simulink subsystem "DCDC_Generator"  (R2024a)
settings: Solver=VariableStepAuto  StartTime=0.0  StopTime=10.0  RelTol=1e-3
undefined symbols (not defined in the file): eta_conv, eta_rect, R_rect, V_drop
settings Model: Creator=User  LastModifiedBy=User

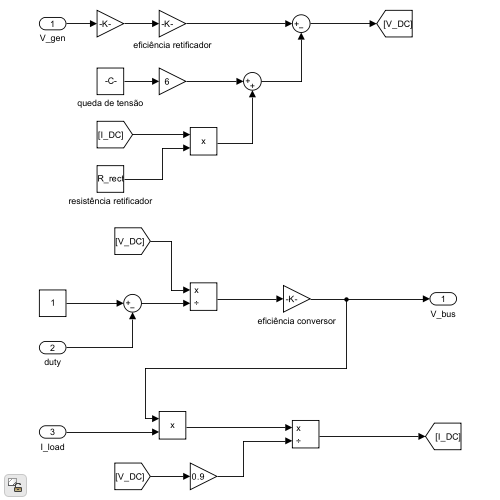
[thumbnail: Simulink's stored preview of the top-level diagram]
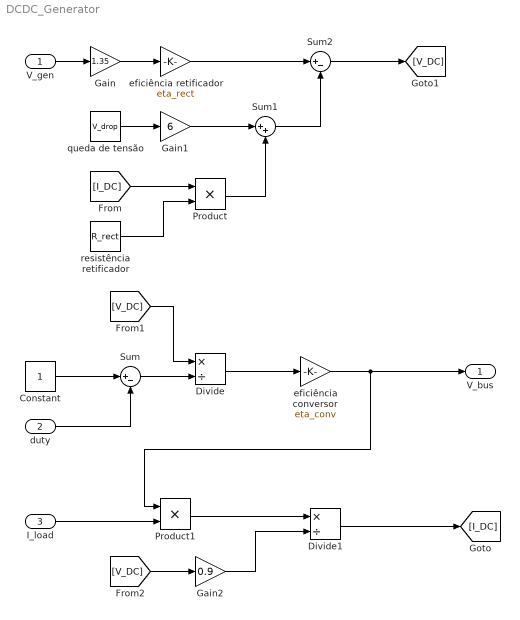
== system DCDC_Generator ==
  V_gen : Inport
  duty : Inport  Port=2
  I_load : Inport  Port=3
  Constant : Constant
  Divide : Product  Inputs=*/
  Divide1 : Product  Inputs=*/
  Gain : Gain  Gain=1.35
  Gain1 : Gain  Gain=6
  Gain2 : Gain  Gain=0.9
  Product : Product
  Product1 : Product
  Sum : Sum  Inputs=|+-
  Sum1 : Sum  Inputs=|++
  Sum2 : Sum  Inputs=|+-
  eficiência conversor : Gain  Gain=eta_conv
  eficiência retificador : Gain  Gain=eta_rect
  queda de tensão : Constant  Value=V_drop
  resistência retificador : Constant  Value=R_rect
  V_bus : Outport
  wires:
  V_gen/1 -> Gain/1
  Constant/1 -> Sum/1
  duty/1 -> Sum/2
  Sum/1 -> Divide/2
  Divide/1 -> eficiência conversor/1
  queda de tensão/1 -> Gain1/1
  [I_DC] -> Product/1
  resistência retificador/1 -> Product/2
  Gain1/1 -> Sum1/1
  Product/1 -> Sum1/2
  Gain/1 -> eficiência retificador/1
  Sum1/1 -> Sum2/2
  eficiência retificador/1 -> Sum2/1
  Sum2/1 -> [V_DC]
  [V_DC] -> Divide/1
  eficiência conversor/1 -> Product1/1, V_bus/1
  I_load/1 -> Product1/2
  Product1/1 -> Divide1/1
  Divide1/1 -> [I_DC]
  [V_DC] -> Gain2/1
  Gain2/1 -> Divide1/2
